simulink model "lab5servo"  (Simulink 7.1)
settings: Solver=ode45  StartTime=0.0  StopTime=10.0  RelTol=1e-3
libraries: simulink x1
settings Model: Creator=ALUNO  LastModifiedBy=ALUNO

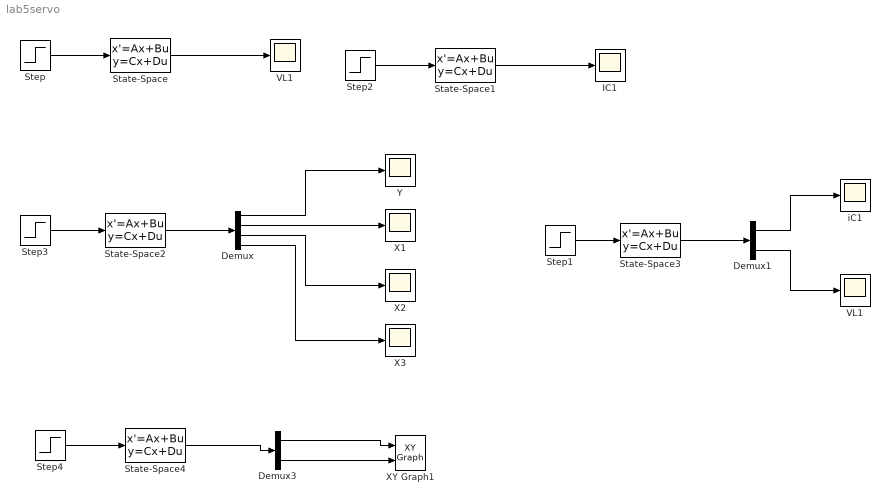
== system lab5servo ==
  Demux : Demux
  Demux1 : Demux  Outputs=2
  Demux3 : Demux  Outputs=2
  IC1 : Scope
      settings: SaveName=ScopeData6
  State-Space : StateSpace  A=[-4 0 -2; 0 -4 1; 8/3 -8/3 0]  B=[2;0;0]  C=[-2 0 -1]
  State-Space1 : StateSpace  A=[-4 0 -2; 0 -4 1; 8/3 -8/3 0]  B=[2;0;0]  C=[1 -1 0]  D=0
  State-Space2 : StateSpace  A=[-4 0 -2; 0 -4 1; 8/3 -8/3 0]  B=[2;0;0]  C=[0 4 0; 1 0 0; 0 1 0; 0 0 1]  D=[0 ; 0; 0; 0]
  State-Space3 : StateSpace  A=[-4 0 -2; 0 -4 1; 8/3 -8/3 0]  B=[2;0;0]  C=[1 -1 0; -2 0 -1]  D=[0 ; 1]
  State-Space4 : StateSpace  A=[-4 2; -3 1]  B=[0 ; 0]  C=[1 0; 0 1]  D=[0 ; 0]  X0=[4; -5]
  Step{,1..4} (5 alike) : Step  Time=0  SampleTime=0
  VL1 : Scope
      settings: SaveName=ScopeData5
  "VL1 " : Scope
  X1 : Scope
      settings: SaveName=ScopeData2
  X2 : Scope
      settings: SaveName=ScopeData3
  X3 : Scope
      settings: SaveName=ScopeData4
  XY Graph1 : simulink/Sinks/XY Graph  SystemSampleTime=-1  xmin=-5  xmax=5  ymin=-5  ymax=5  st=-1
  Y : Scope
  iC1 : Scope
      settings: SaveName=ScopeData10
  wires:
  Step/1 -> State-Space/1
  State-Space/1 -> "VL1 "/1
  Step3/1 -> State-Space2/1
  State-Space2/1 -> Demux/1
  Demux/1 -> Y/1
  Demux/2 -> X1/1
  Demux/3 -> X2/1
  Demux/4 -> X3/1
  Step1/1 -> State-Space3/1
  State-Space3/1 -> Demux1/1
  Demux1/1 -> iC1/1
  Demux1/2 -> VL1/1
  Step2/1 -> State-Space1/1
  State-Space1/1 -> IC1/1
  Step4/1 -> State-Space4/1
  Demux3/1 -> XY Graph1/1
  Demux3/2 -> XY Graph1/2
  State-Space4/1 -> Demux3/1
